simulink model "ex2a_linearized"  (R2020a)
settings: Solver=VariableStepAuto  StartTime=0.0  StopTime=100.0  RelTol=1e-3
settings Model: Creator=mumun  LastModifiedBy=mumun

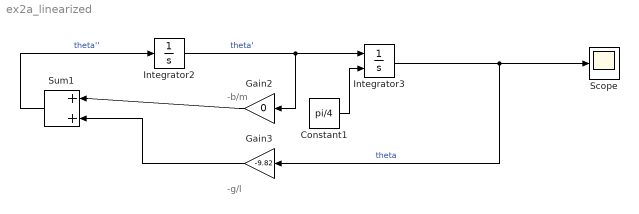
== system ex2a_linearized ==
  note: -g/l
  note: -b/m
  Constant1 : Constant  Value=pi/4
  Gain2 : Gain  Gain=0
  Gain3 : Gain  Gain=-9.82
  Integrator2 : Integrator
  Integrator3 : Integrator  InitialConditionSource=external
  Scope : Scope
  Sum1 : Sum  Inputs=|++
  wires:
  Gain2/1 -> Sum1/1
  Gain3/1 -> Sum1/2
  Constant1/1 -> Integrator3/2
  Sum1/1 -> Integrator2/1  "theta''"
  Integrator3/1 -> Scope/1, Gain3/1  "theta"
  Integrator2/1 -> Gain2/1, Integrator3/1  "theta'"
